simulink model "Modelo_completo_ML_observador_reducido"  (R2023b)
settings: Solver=VariableStepAuto  StartTime=0.0  StopTime=1  MaxStep=1e-5  RelTol=1e-3
values from neighbouring files (symbols this model uses):
  alpha_cu = 3.9 * 10^(-3)    (= 0.0039)    [parametros.m]
  b_eq = 2.1944e-5    (= 2.1944e-05)    [diagrama_polos_y_ceros_LTI.m]    (also in main.m = 2.19444444444e-05; parametros.m = 2.19444444444e-05)
  C_ts = 0.818    [parametros.m]
  J_eq = 1.9785e-5    (= 1.9785e-05)    [diagrama_polos_y_ceros_LTI.m]    (also in main.m = 1.97847222222e-05; parametros.m = 1.97847222222e-05)
  k_l = 0.25    [main.m]    (also in parametros.m)
  P_p = 3    [diagrama_polos_y_ceros_LTI.m]    (also in main.m; parametros.m; variacion_de_parametros.m)
  r = 120.0    (= 120)    [diagrama_polos_y_ceros_LTI.m]    (also in main.m; parametros.m)
  R_sref = 1.02    [parametros.m]
  R_tsamb = 146.7    [parametros.m]
  T_sref = 20    [parametros.m]
settings Model: Creator=nicol  LastModifiedBy=nicol

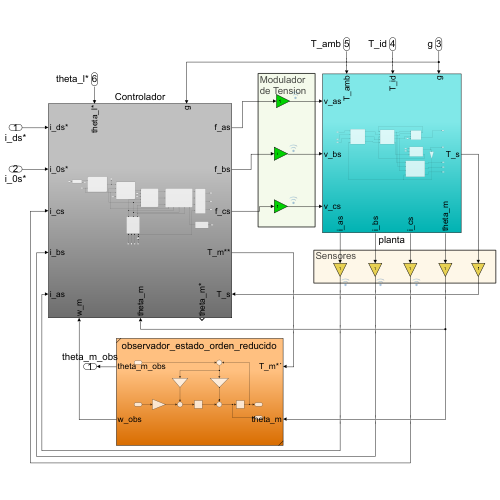
[thumbnail: Simulink's stored preview of the top-level diagram]
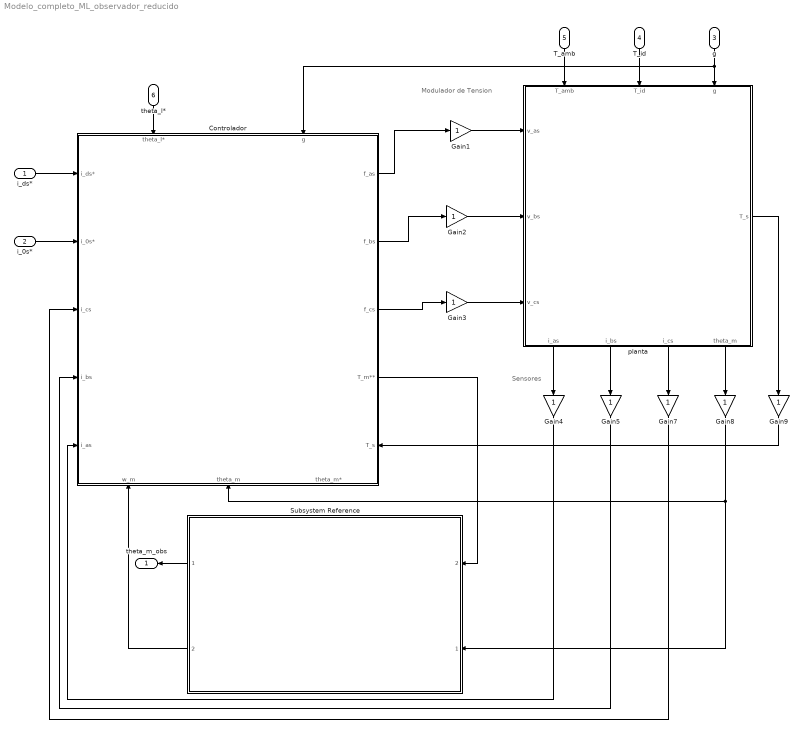
== system Modelo_completo_ML_observador_reducido ==
  note: Sensores
  note: Modulador
      | de Tension
  i_ds* : Inport
  i_0s* : Inport  Port=2
  g : Inport  Port=3
  T_id : Inport  Port=4
  T_amb : Inport  Port=5
  theta_l* : Inport  Port=6
  Controlador : Subsystem
      settings: PortSchema="{\"entries\":[{\"content\":{\"sides\":[{\"content\":{\"connectorIds\":[\"In1\",\"In2\",\"In3\",\"In4\",\"In5\"]},\"type\":\"ConnectorPlacement.EquallySpacedRectSide\",\"uuid\":\"3b7509b8-35e3-46e6-a4cf-9cdf198da4d2\"},{\"content\":{\"connectorIds\":[\"Out1\",\"Out2\",\"Out3\",\"Out4\",\"In10\"],\"side\":\"RIGHT\"},\"type\":\"ConnectorPlacement.EquallySpacedRectSide\",\"uuid\":\"73d58d7e-46e5-46d0-9309-7a6f19fbd3ce\"},{\"content\":{\"connectorIds\":[\"In6\",\"In7\"],\"side\":\"TOP\"},\"type\":\"ConnectorPlacement.EquallySpacedRectSide\",\"uuid\":\"d6185aa2-a2ba-4d2a-9f03-1bc758fc9281\"},{\"content\":{\"connectorIds\":[\"In8\",\"In9\",\"Out5\"],\"side\":\"BOTTOM\"},\"type\":\"ConnectorPlacement.EquallySpacedRectSide\",\"uuid\":\"53443e68-5360-4252-adef-0249763e7699\"}]},\"type\":\"ConnectorPlacement.EquallySpacedConnector\",\"uuid\":\"d42895ef-8e86-49d4-ae05-16f60be7a88b\"}],\"packageUris\":[\"http://schema.mathworks.com/mf0/Connector/R2020b\"],\"version\":\"1.0\"}"
  Gain{1..5,7..9} (8 alike) : Gain
  Subsystem Reference : Subsystem  ReferencedSubsystem=observador_estado_orden_reducido
      settings: PortSchema="{\"entries\":[{\"content\":{\"sides\":[{\"content\":{\"connectorIds\":[\"In2\",\"In1\"]},\"type\":\"ConnectorPlacement.EquallySpacedRectSide\",\"uuid\":\"ff56feed-726a-4eaa-9f54-0c5cb281c862\"},{\"content\":{\"connectorIds\":[\"Out1\",\"Out2\"],\"side\":\"RIGHT\"},\"type\":\"ConnectorPlacement.EquallySpacedRectSide\",\"uuid\":\"814bc364-86f0-4c8e-a19d-b8f51d4e2eb4\"},{\"content\":{\"side\":\"TOP\"},\"type\":\"ConnectorPlacement.EquallySpacedRectSide\",\"uuid\":\"c58d9663-6385-4184-96a5-c81a32fadd7c\"}]},\"type\":\"ConnectorPlacement.EquallySpacedConnector\",\"uuid\":\"f4819058-808d-48e3-ae45-c2f2c77a1307\"}],\"packageUris\":[\"http://schema.mathworks.com/mf0/Connector/R2020b\"],\"version\":\"1.0\"}"
  planta : Subsystem
      settings: PortSchema="{\"entries\":[{\"content\":{\"sides\":[{\"content\":{\"connectorIds\":[\"In1\",\"In2\",\"In3\"]},\"type\":\"ConnectorPlacement.EquallySpacedRectSide\",\"uuid\":\"2cf6e661-0430-4ac8-a786-dfa08ffeeb54\"},{\"content\":{\"connectorIds\":[\"Out1\"],\"side\":\"RIGHT\"},\"type\":\"ConnectorPlacement.EquallySpacedRectSide\",\"uuid\":\"d76a4f35-fdbe-4ab9-8127-b0e4effef06c\"},{\"content\":{\"connectorIds\":[\"In4\",\"In5\",\"In6\"],\"side\":\"TOP\"},\"type\":\"ConnectorPlacement.EquallySpacedRectSide\",\"uuid\":\"e280a4ce-2875-4086-a9ae-a62a28e40d14\"},{\"content\":{\"connectorIds\":[\"Out2\",\"Out3\",\"Out4\",\"Out5\"],\"side\":\"BOTTOM\"},\"type\":\"ConnectorPlacement.EquallySpacedRectSide\",\"uuid\":\"3ec764cb-1cf8-4a25-8759-cfccbcca4007\"}]},\"type\":\"ConnectorPlacement.EquallySpacedConnector\",\"uuid\":\"124f73b6-a202-4770-9cb1-4c0d62f02b41\"}],\"packageUris\":[\"http://schema.mathworks.com/mf0/Connector/R2020b\"],\"version\":\"1.0\"}"
  theta_m_obs : Outport
  wires:
  planta/2(i_as) -> Gain4/1
  planta/3(i_bs) -> Gain5/1
  planta/4(i_cs) -> Gain7/1
  planta/5(theta_m) -> Gain8/1
  planta/1(T_s) -> Gain9/1
  Gain1/1 -> planta/1(v_as)
  Gain2/1 -> planta/2(v_bs)
  Gain3/1 -> planta/3(v_cs)
  Controlador/1(f_as) -> Gain1/1
  Controlador/2(f_bs) -> Gain2/1
  Controlador/3(f_cs) -> Gain3/1
  i_ds*/1 -> Controlador/1(i_ds*)
  i_0s*/1 -> Controlador/2(i_0s*)
  Subsystem Reference/2 -> Controlador/8(w_m)
  Gain8/1 -> Subsystem Reference/1, Controlador/9(theta_m)
  Controlador/4(T_m**) -> Subsystem Reference/2
  Gain9/1 -> Controlador/10(T_s)
  g/1 -> planta/6(g), Controlador/7(g)
  T_id/1 -> planta/5(T_id)
  T_amb/1 -> planta/4(T_amb)
  Subsystem Reference/1 -> theta_m_obs/1
  Gain4/1 -> Controlador/5(i_as)
  Gain5/1 -> Controlador/4(i_bs)
  Gain7/1 -> Controlador/3(i_cs)
  theta_l*/1 -> Controlador/6(theta_l*)

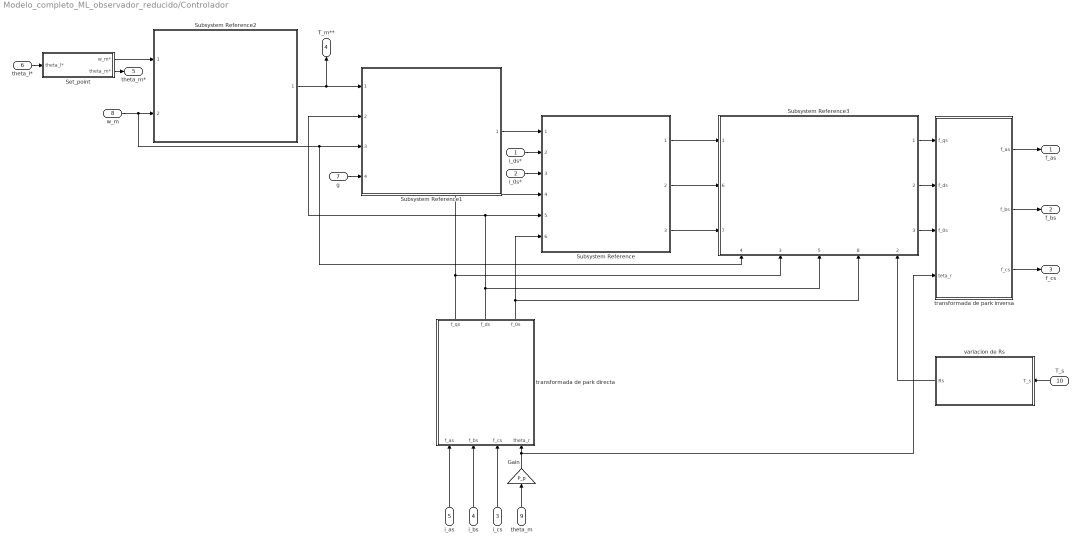
== system Modelo_completo_ML_observador_reducido/Controlador ==
  i_ds* : Inport
  i_0s* : Inport  Port=2
  i_cs : Inport  Port=3
  i_bs : Inport  Port=4
  i_as : Inport  Port=5
  theta_l* : Inport  Port=6
  g : Inport  Port=7
  w_m : Inport  Port=8
  theta_m : Inport  Port=9
  T_s : Inport  Port=10
  Gain : Gain  Gain=P_p
  Set_point : Subsystem
  Subsystem Reference : Subsystem  ReferencedSubsystem=lazo_control_corriente
  Subsystem Reference1 : Subsystem  ReferencedSubsystem=consigna_torque_y_compensaciones
  Subsystem Reference2 : Subsystem  ReferencedSubsystem=controlador_posicion_velocidad
  Subsystem Reference3 : Subsystem  ReferencedSubsystem=desacople_realimentacion_fisicas_naturales
      settings: PortSchema="{\"entries\":[{\"content\":{\"sides\":[{\"content\":{\"connectorIds\":[\"In1\",\"In6\",\"In7\"]},\"type\":\"ConnectorPlacement.EquallySpacedRectSide\",\"uuid\":\"c16960c1-ac00-4f2f-b262-353f165eb751\"},{\"content\":{\"connectorIds\":[\"Out1\",\"Out2\",\"Out3\"],\"side\":\"RIGHT\"},\"type\":\"ConnectorPlacement.EquallySpacedRectSide\",\"uuid\":\"8f19cbef-98ae-4dfe-90e9-8b934adc47d9\"},{\"content\":{\"side\":\"TOP\"},\"type\":\"ConnectorPlacement.EquallySpacedRectSide\",\"uuid\":\"a2a080d0-f29c-409f-9d43-6daa49356984\"},{\"content\":{\"connectorIds\":[\"In4\",\"In3\",\"In5\",\"In8\",\"In2\"],\"side\":\"BOTTOM\"},\"type\":\"ConnectorPlacement.EquallySpacedRectSide\",\"uuid\":\"36e587f2-4d9a-4522-abd7-5d6009ea3dc1\"}]},\"type\":\"ConnectorPlacement.EquallySpacedConnector\",\"uuid\":\"857f20c7-d01e-4fb7-9a94-d371d298e7ea\"}],\"packageUris\":[\"http://schema.mathworks.com/mf0/Connector/R2020b\"],\"version\":\"1.0\"}"
  transformada de park directa : Subsystem
  transformada de park inversa : Subsystem
  variacion de Rs : Subsystem
  f_as : Outport
  f_bs : Outport  Port=2
  f_cs : Outport  Port=3
  T_m** : Outport  Port=4
  theta_m* : Outport  Port=5
  wires:
  Subsystem Reference1/1 -> Subsystem Reference/1
  Subsystem Reference2/1 -> Subsystem Reference1/1, T_m**/1
  Subsystem Reference3/2 -> transformada de park inversa/2(f_ds)
  Subsystem Reference3/1 -> transformada de park inversa/1(f_qs)
  Subsystem Reference3/3 -> transformada de park inversa/3(f_0s)
  Subsystem Reference/1 -> Subsystem Reference3/1
  Subsystem Reference/2 -> Subsystem Reference3/6
  Subsystem Reference/3 -> Subsystem Reference3/7
  variacion de Rs/1(Rs) -> Subsystem Reference3/2
  i_ds*/1 -> Subsystem Reference/2
  i_0s*/1 -> Subsystem Reference/3
  transformada de park directa/3(f_0s) -> Subsystem Reference3/8, Subsystem Reference/6
  transformada de park directa/2(f_ds) -> Subsystem Reference3/5, Subsystem Reference1/2, Subsystem Reference/5
  transformada de park directa/1(f_qs) -> Subsystem Reference3/3, Subsystem Reference/4
  transformada de park inversa/1(f_as) -> f_as/1
  transformada de park inversa/2(f_bs) -> f_bs/1
  transformada de park inversa/3(f_cs) -> f_cs/1
  i_as/1 -> transformada de park directa/1(f_as)
  i_bs/1 -> transformada de park directa/2(f_bs)
  i_cs/1 -> transformada de park directa/3(f_cs)
  w_m/1 -> Subsystem Reference2/2, Subsystem Reference3/4, Subsystem Reference1/3
  g/1 -> Subsystem Reference1/4
  T_s/1 -> variacion de Rs/1(T_s)
  Set_point/1(w_m*) -> Subsystem Reference2/1
  theta_l*/1 -> Set_point/1(theta_l*)
  Set_point/2(theta_m*) -> theta_m*/1
  theta_m/1 -> Gain/1
  Gain/1 -> transformada de park inversa/4(teta_r), transformada de park directa/4(theta_r)

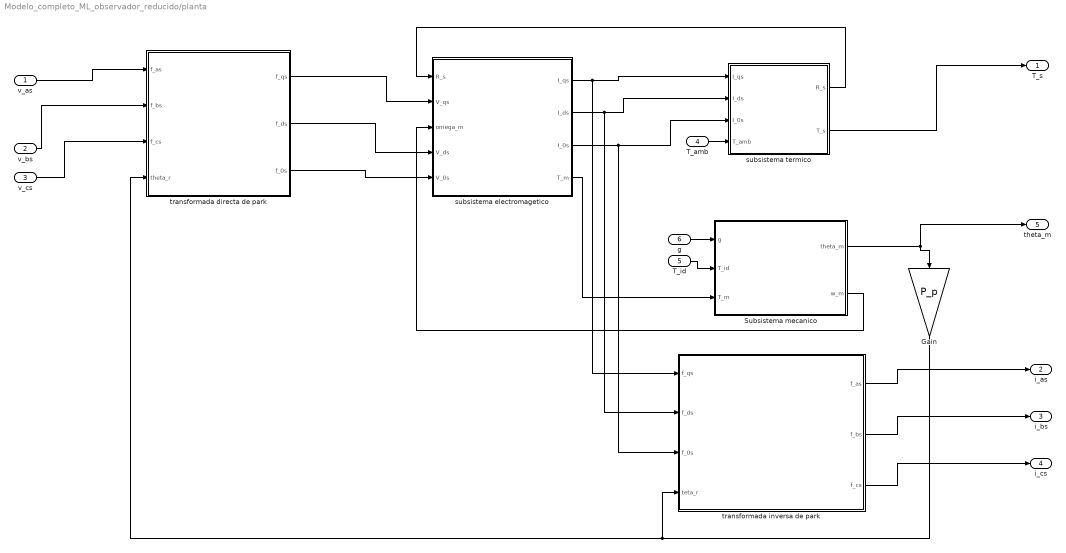
== system Modelo_completo_ML_observador_reducido/planta ==
  v_as : Inport
  v_bs : Inport  Port=2
  v_cs : Inport  Port=3
  T_amb : Inport  Port=4
  T_id : Inport  Port=5
  g : Inport  Port=6
  Gain : Gain  Gain=P_p
  Subsistema mecanico : Subsystem
  subsistema electromagetico : Subsystem
  subsistema termico : Subsystem
  transformada directa de park : Subsystem
  transformada inversa de park : Subsystem
  T_s : Outport
  i_as : Outport  Port=2
  i_bs : Outport  Port=3
  i_cs : Outport  Port=4
  theta_m : Outport  Port=5
  wires:
  g/1 -> Subsistema mecanico/1(g)
  T_id/1 -> Subsistema mecanico/2(T_id)
  T_amb/1 -> subsistema termico/4(T_amb)
  transformada directa de park/1(f_qs) -> subsistema electromagetico/2(V_qs)
  transformada directa de park/2(f_ds) -> subsistema electromagetico/4(V_ds)
  transformada directa de park/3(f_0s) -> subsistema electromagetico/5(V_0s)
  subsistema termico/1(R_s) -> subsistema electromagetico/1(R_s)
  subsistema electromagetico/1(I_qs) -> transformada inversa de park/1(f_qs), subsistema termico/1(I_qs)
  subsistema electromagetico/2(I_ds) -> transformada inversa de park/2(f_ds), subsistema termico/2(I_ds)
  subsistema electromagetico/3(I_0s) -> transformada inversa de park/3(f_0s), subsistema termico/3(I_0s)
  subsistema electromagetico/4(T_m) -> Subsistema mecanico/3(T_m)
  Subsistema mecanico/2(w_m) -> subsistema electromagetico/3(omega_m)
  Subsistema mecanico/1(theta_m) -> theta_m/1, Gain/1
  Gain/1 -> transformada directa de park/4(theta_r), transformada inversa de park/4(teta_r)
  v_as/1 -> transformada directa de park/1(f_as)
  v_bs/1 -> transformada directa de park/2(f_bs)
  v_cs/1 -> transformada directa de park/3(f_cs)
  subsistema termico/2(T_s) -> T_s/1
  transformada inversa de park/1(f_as) -> i_as/1
  transformada inversa de park/2(f_bs) -> i_bs/1
  transformada inversa de park/3(f_cs) -> i_cs/1

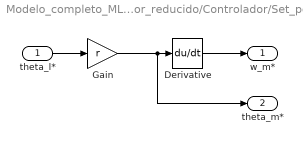
== system Modelo_completo_ML_observador_reducido/Controlador/Set_point ==
  theta_l* : Inport
  Derivative : Derivative
  Gain : Gain  Gain=r
  w_m* : Outport
  theta_m* : Outport  Port=2
  wires:
  Derivative/1 -> w_m*/1
  theta_l*/1 -> Gain/1
  Gain/1 -> theta_m*/1, Derivative/1

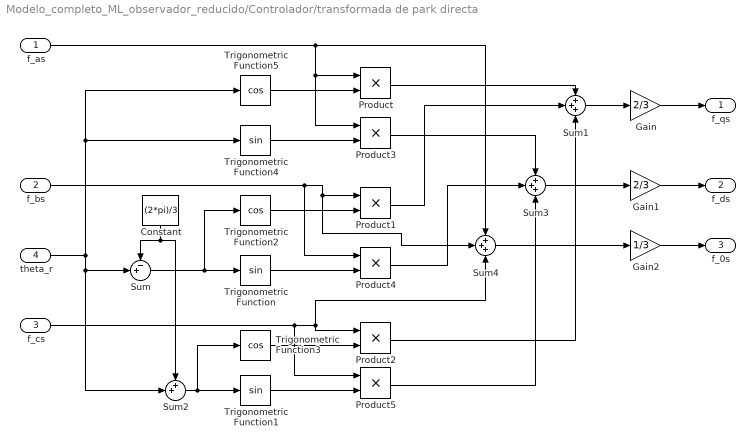
== system Modelo_completo_ML_observador_reducido/Controlador/transformada de park directa ==
  f_as : Inport
  f_bs : Inport  Port=2
  f_cs : Inport  Port=3
  theta_r : Inport  Port=4
  Constant : Constant  Value=(2*pi)/3
  Gain : Gain  Gain=2/3
  Gain1 : Gain  Gain=2/3
  Gain2 : Gain  Gain=1/3
  Product{,1..5} (6 alike) : Product
  Sum : Sum  Inputs=-+|
  Sum1 : Sum  Inputs=+++
  Sum2 : Sum  Inputs=++|
  Sum3 : Sum  Inputs=+++
  Sum4 : Sum  Inputs=+++
  Trigonometric Function : Trigonometry
  Trigonometric Function1 : Trigonometry
  Trigonometric Function2 : Trigonometry  Operator=cos
  Trigonometric Function3 : Trigonometry  Operator=cos
  Trigonometric Function4 : Trigonometry
  Trigonometric Function5 : Trigonometry  Operator=cos
  f_qs : Outport
  f_ds : Outport  Port=2
  f_0s : Outport  Port=3
  wires:
  f_cs/1 -> Sum4/3, Product2/1, Product5/1
  Product2/1 -> Sum1/3
  f_as/1 -> Sum4/1, Product3/1, Product/1
  Product3/1 -> Sum3/1
  Product5/1 -> Sum3/3
  Sum2/1 -> Trigonometric Function3/1, Trigonometric Function1/1
  Product4/1 -> Sum3/2
  Product1/1 -> Sum1/2
  Sum4/1 -> Gain2/1
  Sum1/1 -> Gain/1
  Trigonometric Function1/1 -> Product5/2
  Constant/1 -> Sum/1, Sum2/1
  Sum/1 -> Trigonometric Function/1, Trigonometric Function2/1
  Trigonometric Function3/1 -> Product2/2
  Trigonometric Function2/1 -> Product1/2
  Gain1/1 -> f_ds/1
  Gain2/1 -> f_0s/1
  Product/1 -> Sum1/1
  Trigonometric Function/1 -> Product4/2
  Gain/1 -> f_qs/1
  theta_r/1 -> Sum2/2, Sum/2, Trigonometric Function5/1, Trigonometric Function4/1
  Trigonometric Function5/1 -> Product/2
  f_bs/1 -> Sum4/2, Product1/1, Product4/1
  Sum3/1 -> Gain1/1
  Trigonometric Function4/1 -> Product3/2

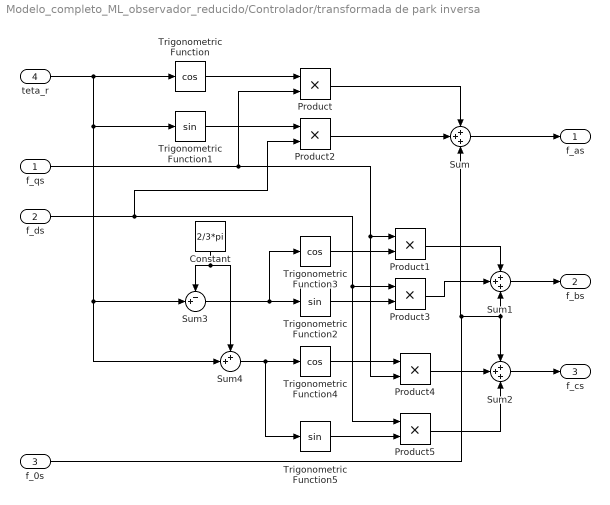
== system Modelo_completo_ML_observador_reducido/Controlador/transformada de park inversa ==
  f_qs : Inport
  f_ds : Inport  Port=2
  f_0s : Inport  Port=3
  teta_r : Inport  Port=4
  Constant : Constant  Value=2/3*pi
  Product{,1..5} (6 alike) : Product
  Sum : Sum  Inputs=+++
  Sum1 : Sum  Inputs=+++
  Sum2 : Sum  Inputs=+++
  Sum3 : Sum  Inputs=-+|
  Sum4 : Sum  Inputs=++|
  Trigonometric Function : Trigonometry  Operator=cos
  Trigonometric Function1 : Trigonometry
  Trigonometric Function2 : Trigonometry
  Trigonometric Function3 : Trigonometry  Operator=cos
  Trigonometric Function4 : Trigonometry  Operator=cos
  Trigonometric Function5 : Trigonometry
  f_as : Outport
  f_bs : Outport  Port=2
  f_cs : Outport  Port=3
  wires:
  f_ds/1 -> Product3/1, Product5/1, Product2/2
  Product5/1 -> Sum2/3
  Product3/1 -> Sum1/2
  Constant/1 -> Sum4/1, Sum3/1
  Sum1/1 -> f_bs/1
  Trigonometric Function5/1 -> Product5/2
  Trigonometric Function2/1 -> Product3/2
  Trigonometric Function4/1 -> Product4/1
  Product4/1 -> Sum2/2
  f_qs/1 -> Product1/1, Product4/2, Product/2
  Sum3/1 -> Trigonometric Function3/1, Trigonometric Function2/1
  Trigonometric Function3/1 -> Product1/2
  Trigonometric Function1/1 -> Product2/1
  f_0s/1 -> Sum/3, Sum2/1, Sum1/3
  teta_r/1 -> Sum4/2, Sum3/2, Trigonometric Function1/1, Trigonometric Function/1
  Product/1 -> Sum/1
  Sum2/1 -> f_cs/1
  Trigonometric Function/1 -> Product/1
  Product2/1 -> Sum/2
  Sum/1 -> f_as/1
  Product1/1 -> Sum1/1
  Sum4/1 -> Trigonometric Function5/1, Trigonometric Function4/1

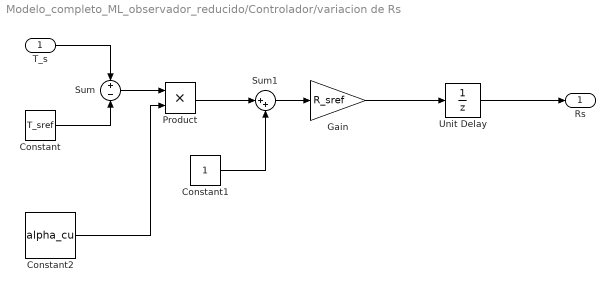
== system Modelo_completo_ML_observador_reducido/Controlador/variacion de Rs ==
  T_s : Inport
  Constant : Constant  Value=T_sref
  Constant1 : Constant
  Constant2 : Constant  Value=alpha_cu
  Gain : Gain  Gain=R_sref
  Product : Product
  Sum : Sum  Inputs=+-
  Sum1 : Sum  Inputs=|++
  Unit Delay : UnitDelay  SampleTime=-1  HasFrameUpgradeWarning=on
  Rs : Outport
  wires:
  T_s/1 -> Sum/1
  Unit Delay/1 -> Rs/1
  Product/1 -> Sum1/1
  Constant/1 -> Sum/2
  Constant2/1 -> Product/2
  Sum1/1 -> Gain/1
  Gain/1 -> Unit Delay/1
  Constant1/1 -> Sum1/2
  Sum/1 -> Product/1

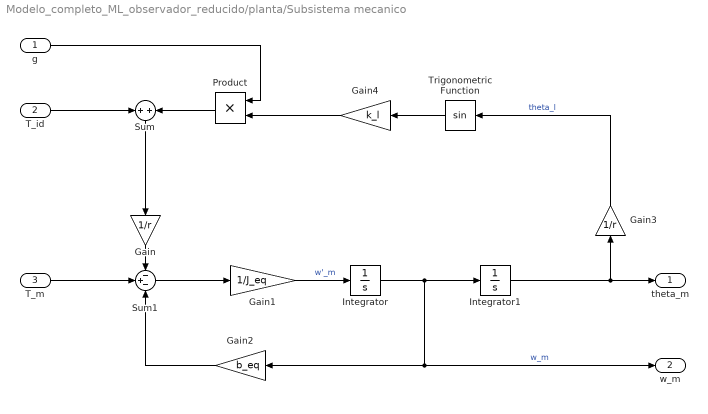
== system Modelo_completo_ML_observador_reducido/planta/Subsistema mecanico ==
  g : Inport
  T_id : Inport  Port=2
  T_m : Inport  Port=3
  Gain : Gain  Gain=1/r
  Gain1 : Gain  Gain=1/J_eq
  Gain2 : Gain  Gain=b_eq
  Gain3 : Gain  Gain=1/r
  Gain4 : Gain  Gain=k_l
  Integrator : Integrator
  Integrator1 : Integrator
  Product : Product
  Sum : Sum
  Sum1 : Sum  Inputs=-+-
  Trigonometric Function : Trigonometry
  theta_m : Outport
  w_m : Outport  Port=2
  wires:
  Sum/1 -> Gain/1
  Sum1/1 -> Gain1/1
  Gain1/1 -> Integrator/1  "w'_m"
  g/1 -> Product/1
  T_m/1 -> Sum1/2
  T_id/1 -> Sum/1
  Gain2/1 -> Sum1/3
  Gain/1 -> Sum1/1
  Integrator/1 -> Integrator1/1, w_m/1, Gain2/1  "w_m"
  Product/1 -> Sum/2
  Gain3/1 -> Trigonometric Function/1  "theta_l"
  Trigonometric Function/1 -> Gain4/1
  Integrator1/1 -> theta_m/1, Gain3/1
  Gain4/1 -> Product/2

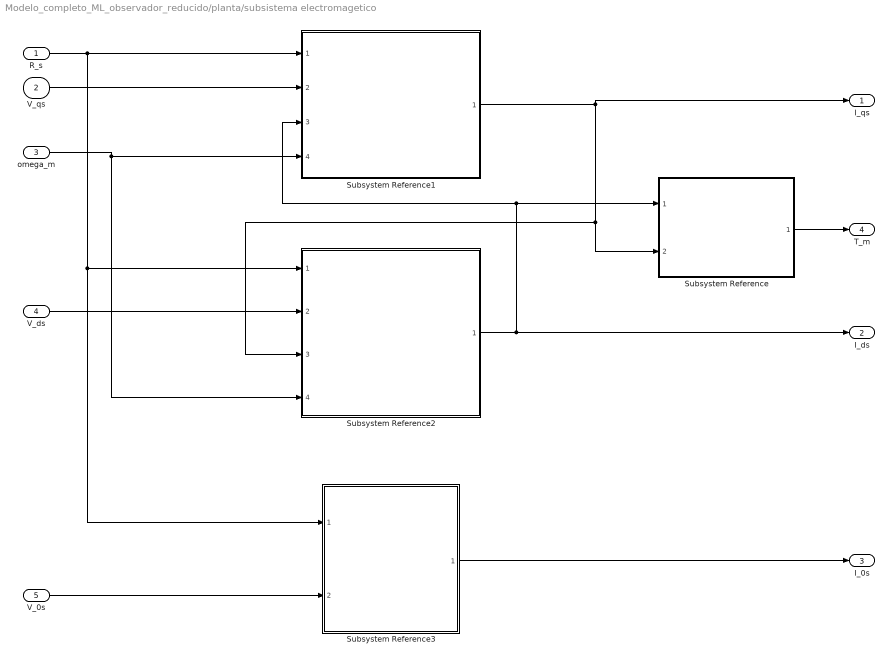
== system Modelo_completo_ML_observador_reducido/planta/subsistema electromagetico ==
  R_s : Inport
  V_qs : Inport  Port=2
  omega_m : Inport  Port=3
  V_ds : Inport  Port=4
  V_0s : Inport  Port=5
  Subsystem Reference : Subsystem  ReferencedSubsystem=subsistema_magnetico_estator
  Subsystem Reference1 : Subsystem  ReferencedSubsystem=subsistema_electrico_corriente_I_qs
  Subsystem Reference2 : Subsystem  ReferencedSubsystem=subsistema_electrico_corriente_I_ds
  Subsystem Reference3 : Subsystem  ReferencedSubsystem=subsistema_electrico_corriente_I_0s
  I_qs : Outport
  I_ds : Outport  Port=2
  I_0s : Outport  Port=3
  T_m : Outport  Port=4
  wires:
  Subsystem Reference/1 -> T_m/1
  V_ds/1 -> Subsystem Reference2/2
  omega_m/1 -> Subsystem Reference1/4, Subsystem Reference2/4
  V_0s/1 -> Subsystem Reference3/2
  V_qs/1 -> Subsystem Reference1/2
  Subsystem Reference1/1 -> I_qs/1, Subsystem Reference/2, Subsystem Reference2/3
  Subsystem Reference2/1 -> Subsystem Reference1/3, Subsystem Reference/1, I_ds/1
  Subsystem Reference3/1 -> I_0s/1
  R_s/1 -> Subsystem Reference1/1, Subsystem Reference2/1, Subsystem Reference3/1

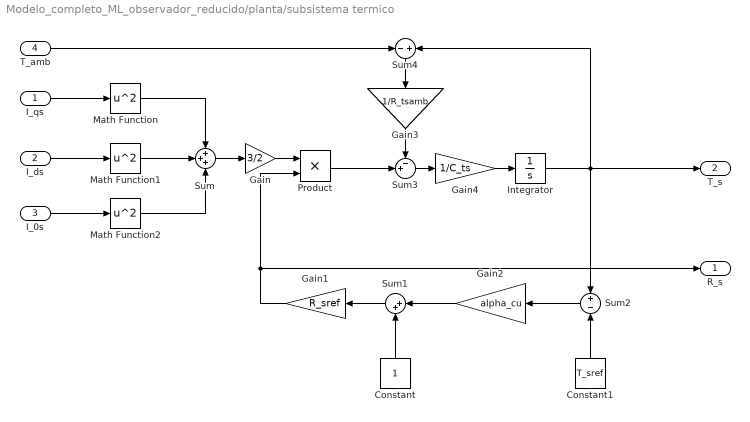
== system Modelo_completo_ML_observador_reducido/planta/subsistema termico ==
  I_qs : Inport
  I_ds : Inport  Port=2
  I_0s : Inport  Port=3
  T_amb : Inport  Port=4
  Constant : Constant
  Constant1 : Constant  Value=T_sref
  Gain : Gain  Gain=3/2
  Gain1 : Gain  Gain=R_sref
  Gain2 : Gain  Gain=alpha_cu
  Gain3 : Gain  Gain=1/R_tsamb
  Gain4 : Gain  Gain=1/C_ts
  Integrator : Integrator  InitialCondition=20
  Math Function : Math  Operator=square
  Math Function1 : Math  Operator=square
  Math Function2 : Math  Operator=square
  Product : Product
  Sum : Sum  Inputs=+++
  Sum1 : Sum  Inputs=|++
  Sum2 : Sum  Inputs=+|-
  Sum3 : Sum  Inputs=-+|
  Sum4 : Sum  Inputs=-|+
  R_s : Outport
  T_s : Outport  Port=2
  wires:
  Gain1/1 -> Product/2, R_s/1
  Constant1/1 -> Sum2/2
  Math Function/1 -> Sum/1
  Gain2/1 -> Sum1/1
  Integrator/1 -> Sum2/1, T_s/1, Sum4/2
  Constant/1 -> Sum1/2
  Gain3/1 -> Sum3/1
  T_amb/1 -> Sum4/1
  Product/1 -> Sum3/2
  Sum3/1 -> Gain4/1
  Gain/1 -> Product/1
  Sum2/1 -> Gain2/1
  I_0s/1 -> Math Function2/1
  Gain4/1 -> Integrator/1
  I_ds/1 -> Math Function1/1
  Sum4/1 -> Gain3/1
  Math Function1/1 -> Sum/2
  Sum/1 -> Gain/1
  I_qs/1 -> Math Function/1
  Sum1/1 -> Gain1/1
  Math Function2/1 -> Sum/3

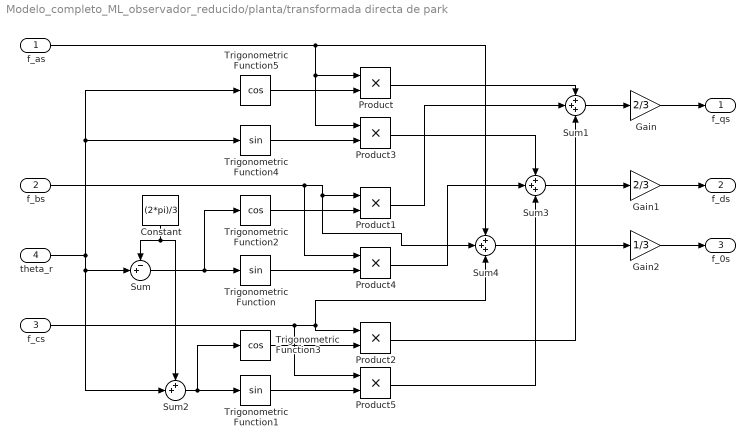
== system Modelo_completo_ML_observador_reducido/planta/transformada directa de park ==
  f_as : Inport
  f_bs : Inport  Port=2
  f_cs : Inport  Port=3
  theta_r : Inport  Port=4
  Constant : Constant  Value=(2*pi)/3
  Gain : Gain  Gain=2/3
  Gain1 : Gain  Gain=2/3
  Gain2 : Gain  Gain=1/3
  Product{,1..5} (6 alike) : Product
  Sum : Sum  Inputs=-+|
  Sum1 : Sum  Inputs=+++
  Sum2 : Sum  Inputs=++|
  Sum3 : Sum  Inputs=+++
  Sum4 : Sum  Inputs=+++
  Trigonometric Function : Trigonometry
  Trigonometric Function1 : Trigonometry
  Trigonometric Function2 : Trigonometry  Operator=cos
  Trigonometric Function3 : Trigonometry  Operator=cos
  Trigonometric Function4 : Trigonometry
  Trigonometric Function5 : Trigonometry  Operator=cos
  f_qs : Outport
  f_ds : Outport  Port=2
  f_0s : Outport  Port=3
  wires:
  Sum4/1 -> Gain2/1
  Sum3/1 -> Gain1/1
  Trigonometric Function3/1 -> Product2/2
  Gain1/1 -> f_ds/1
  Gain2/1 -> f_0s/1
  f_bs/1 -> Sum4/2, Product1/1, Product4/1
  f_as/1 -> Sum4/1, Product3/1, Product/1
  Trigonometric Function2/1 -> Product1/2
  Trigonometric Function4/1 -> Product3/2
  Trigonometric Function/1 -> Product4/2
  Sum/1 -> Trigonometric Function/1, Trigonometric Function2/1
  Gain/1 -> f_qs/1
  Product5/1 -> Sum3/3
  Product3/1 -> Sum3/1
  Trigonometric Function1/1 -> Product5/2
  Product4/1 -> Sum3/2
  Product/1 -> Sum1/1
  theta_r/1 -> Sum2/2, Sum/2, Trigonometric Function5/1, Trigonometric Function4/1
  Constant/1 -> Sum/1, Sum2/1
  Sum2/1 -> Trigonometric Function3/1, Trigonometric Function1/1
  Sum1/1 -> Gain/1
  Product1/1 -> Sum1/2
  f_cs/1 -> Sum4/3, Product2/1, Product5/1
  Product2/1 -> Sum1/3
  Trigonometric Function5/1 -> Product/2

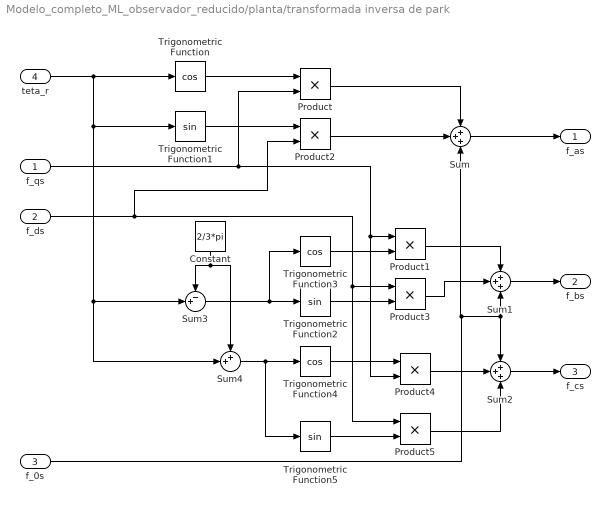
== system Modelo_completo_ML_observador_reducido/planta/transformada inversa de park ==
  f_qs : Inport
  f_ds : Inport  Port=2
  f_0s : Inport  Port=3
  teta_r : Inport  Port=4
  Constant : Constant  Value=2/3*pi
  Product{,1..5} (6 alike) : Product
  Sum : Sum  Inputs=+++
  Sum1 : Sum  Inputs=+++
  Sum2 : Sum  Inputs=+++
  Sum3 : Sum  Inputs=-+|
  Sum4 : Sum  Inputs=++|
  Trigonometric Function : Trigonometry  Operator=cos
  Trigonometric Function1 : Trigonometry
  Trigonometric Function2 : Trigonometry
  Trigonometric Function3 : Trigonometry  Operator=cos
  Trigonometric Function4 : Trigonometry  Operator=cos
  Trigonometric Function5 : Trigonometry
  f_as : Outport
  f_bs : Outport  Port=2
  f_cs : Outport  Port=3
  wires:
  Product1/1 -> Sum1/1
  Sum4/1 -> Trigonometric Function5/1, Trigonometric Function4/1
  Sum2/1 -> f_cs/1
  Product2/1 -> Sum/2
  Trigonometric Function/1 -> Product/1
  Product4/1 -> Sum2/2
  Sum1/1 -> f_bs/1
  Trigonometric Function3/1 -> Product1/2
  Trigonometric Function5/1 -> Product5/2
  Product/1 -> Sum/1
  Sum3/1 -> Trigonometric Function3/1, Trigonometric Function2/1
  Trigonometric Function4/1 -> Product4/1
  f_0s/1 -> Sum/3, Sum2/1, Sum1/3
  Trigonometric Function2/1 -> Product3/2
  f_qs/1 -> Product1/1, Product4/2, Product/2
  teta_r/1 -> Sum4/2, Sum3/2, Trigonometric Function1/1, Trigonometric Function/1
  Product3/1 -> Sum1/2
  Trigonometric Function1/1 -> Product2/1
  f_ds/1 -> Product3/1, Product5/1, Product2/2
  Product5/1 -> Sum2/3
  Constant/1 -> Sum4/1, Sum3/1
  Sum/1 -> f_as/1
